simulink model "oldVers_1704_old1"  (R2022a)
settings: Solver=ode1  StartTime=0.0  StopTime=0.008  FixedStep=0.000001  RelTol=1e-3
values from neighbouring files (symbols this model uses):
  Cm = 0.05    [matlab2.mat]
  Jm = 1    [matlab2.mat]
  k_eq = 1    [matlab2.mat]
  k_pos = 1    [matlab2.mat]
  Ki_Curr = 1666    [matlab2.mat]
  Kinv = 18    [matlab2.mat]
  Kp_Curr = 0.0229017    [matlab2.mat]
  Re = 0.357267    [matlab2.mat]
  T_eq = 0.00052    [matlab2.mat]
  T_eq2 = 0.0018    [matlab2.mat]
  Te = 0.0006    [matlab2.mat]
  Tinv = 0.00026    [matlab2.mat]
undefined symbols (not defined in the file or in its folder): Kc_Curr, Kc_Pos, Kc_Speed
libraries: simulink x1
settings Model: Creator=Ruslan  LastModifiedBy=Ruslan
settings SolverCC: AlgebraicLoopSolver=TrustRegion
settings DebuggingCC: SFMachineParentedDataDiag=warning

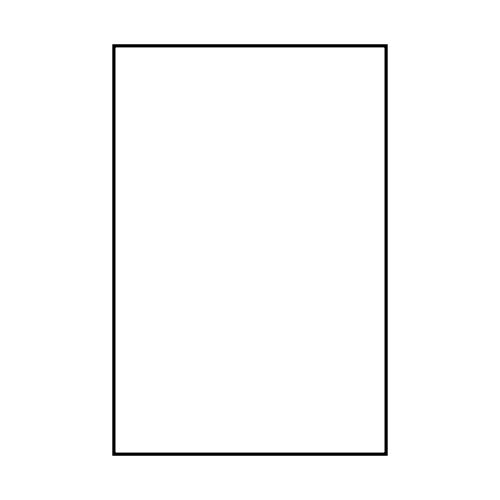
[thumbnail: Simulink's stored preview of the top-level diagram]
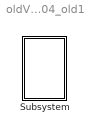
== system oldVers_1704_old1 ==
  Subsystem : Subsystem

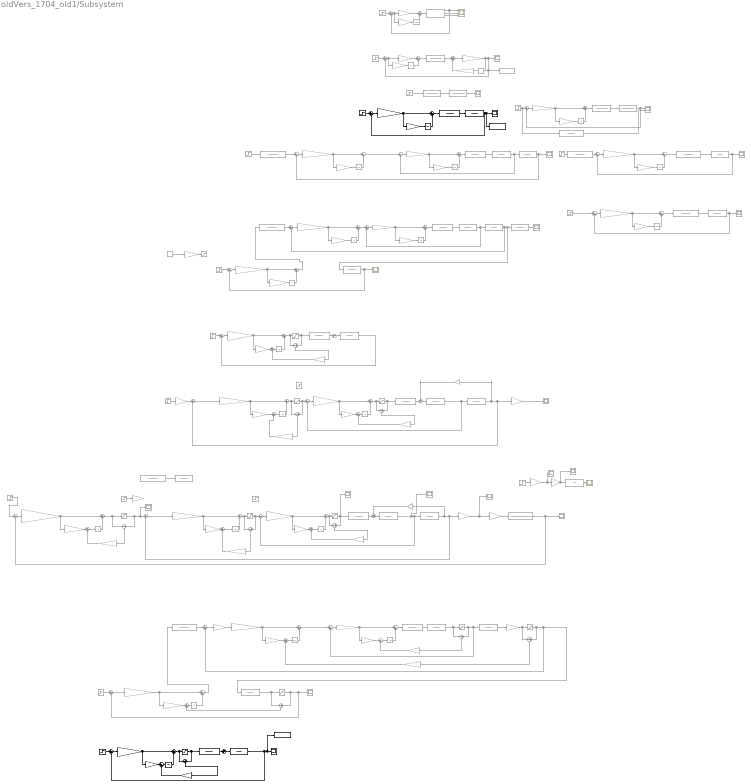
== system oldVers_1704_old1/Subsystem ==
  note: Рабочий Контур скорости с насыщениями
  note: Контур положения рабочий
  note: Контур скорости
  note: Контур тока
  note: Контур тока
  note: Контур тока рабочий
  1 : TransferFcn  Commented=on  Numerator=[Cm]  Denominator=[Jm 0]
  1/Rяц : Gain  Commented=on  Gain=1/0.357267
  {2..5} (4 alike) : TransferFcn  Commented=on  Numerator=[k_pos]  Denominator=[1 0]
  Derivative : Derivative  Commented=on
  Gain : Gain  Commented=on  Gain=Cm
  Gain1 : Gain  Commented=on  Gain=Cm
  Gain2 : Gain  Commented=on  Gain=k_pos*3.33333333333
  Integrator{,1,3..11,13..15,17,19..22} (19 alike) : Integrator  Commented=on
  Integrator12 : Integrator
  Integrator2 : Integrator
  Kп : Gain  Commented=on  Gain=0.00067
  Kп1 : Gain  Commented=on  Gain=0.00067
  Kп{4,7,10,14,17,30} (6 alike) : Gain  Commented=on  Gain=(Jm)/(2*T_eq*Cm)
  Kп11 : Gain  Commented=on  Gain=(1)/(2*T_eq2*k_pos)
  Kп12 : Gain  Commented=on  Gain=Te/(2*Tinv*Kinv*(1/Re))
  Kп13 : Gain  Commented=on  Gain=Kp_Curr
  Kп{15,18,20,26,31} (5 alike) : Gain  Commented=on  Gain=1/(30/pi)
  Kп16 : Gain  Commented=on  Gain=30/pi
  Kп19 : Gain  Commented=on  Gain=Te/(2*Tinv*Kinv*(1/Re))
  Kп2 : Gain  Commented=on  Gain=30/pi
  Kп21 : Gain  Gain=Te/(2*Tinv*Kinv*(1/Re))
  Kп25 : Gain  Commented=on  Gain=(0.06)/(2*T_eq2*k_pos*3.33333333333)
  Kп27 : Gain  Commented=on  Gain=(1)/(2*T_eq2*k_pos)
  Kп28 : Gain  Commented=on  Gain=Kp_Curr
  Kп29 : Gain  Commented=on  Gain=30/pi
  Kп3 : Gain  Commented=on  Gain=Kp_Curr
  Kп5 : Gain  Commented=on  Gain=0.0229017
  Kп6 : Gain  Commented=on  Gain=(1)/(2*T_eq2*k_pos)
  Kп8 : Gain  Gain=Te/(2*Tinv*Kinv*(1/Re))
  Kп9 : Gain  Commented=on  Gain=Te/(2*Tinv*Kinv*(1/Re))
  L : Gain  Commented=on  Gain=0.001457602
  Ramp1 : simulink/Sources/Ramp  Commented=on  slope=120  start=0  InitialOutput=0
  Saturation1 : Saturate  Commented=on  UpperLimit=96  LowerLimit=-40
  Saturation10 : Saturate  Commented=on  UpperLimit=91.6  LowerLimit=-91.6
  Saturation11 : Saturate  Commented=on  UpperLimit=70  LowerLimit=-70
  Saturation12 : Saturate  Commented=on  UpperLimit=1  LowerLimit=-1
  Saturation2 : Saturate  Commented=on  UpperLimit=70  LowerLimit=-70
  Saturation3 : Saturate  Commented=on  UpperLimit=1  LowerLimit=-1
  Saturation4 : Saturate  Commented=on  UpperLimit=1  LowerLimit=-1
  Saturation5 : Saturate  UpperLimit=1  LowerLimit=-1
  Saturation7 : Saturate  Commented=on  UpperLimit=70  LowerLimit=-70
  Saturation8 : Saturate  Commented=on  UpperLimit=750  LowerLimit=-750
  Saturation9 : Saturate  Commented=on  UpperLimit=900  LowerLimit=-900
  Scope : Scope  Commented=on  NumInputPorts=3
  Scope{1..2,4,6..19} (17 alike) : Scope  Commented=on
  Scope20 : Scope
  Scope3 : Scope
  Scope5 : Scope  Commented=on  NumInputPorts=2
  Step : Step  Commented=on  Time=0  After=-12  SampleTime=0
  Step{1..2,4..6,9,13..14} (8 alike) : Step  Commented=on  Time=0  SampleTime=0
  Step10 : Step  Commented=on  Time=0  After=875  SampleTime=0
  Step11 : Step  Commented=on  Time=0  After=96  SampleTime=0
  Step12 : Step  Commented=on  Time=0  After=875  SampleTime=0
  Step15 : Step  Commented=on  Time=0  After=70  SampleTime=0
  Step16 : Step  Commented=on  Time=0  After=18  SampleTime=0
  Step17 : Step  Time=0  After=10  SampleTime=0
  Step3 : Step  Time=0  SampleTime=0
  Step7 : Step  Commented=on  Time=0  After=140  SampleTime=0
  Step8 : Step  Commented=on  Time=0  After=85  SampleTime=0
  Sum{,2,8..9,12,15..16,20,24,27..28,31,35,39,43,51,55,57,61} (19 alike) : Sum  Commented=on  Inputs=|+-
  Sum{1,3,7,10..11,13..14,19,21,23,25..26,30,32,34,36,38,40,42,44,50,53..54,56,58,60,62,65} (28 alike) : Sum  Commented=on  Inputs=|++
  Sum17 : Sum  Commented=on  Inputs=-+|
  Sum18 : Sum  Commented=on  Inputs=-+|
  Sum{22,33,37,41,45,52,59,63..64} (9 alike) : Sum  Commented=on  Inputs=-|+
  Sum29 : Sum  Commented=on  Inputs=-+|
  Sum4 : Sum  Commented=on  Inputs=-+-
  Sum46 : Sum  Inputs=-+|
  Sum47 : Sum  Inputs=|++
  Sum48 : Sum  Inputs=|+-
  Sum49 : Sum  Inputs=|++
  Sum5 : Sum  Inputs=|++
  Sum6 : Sum  Inputs=|+-
  Sum66 : Sum  Inputs=-|+
  To Workspace : ToWorkspace  Commented=on  VariableName=simout  SaveFormat=Timeseries  SampleTime=-1
  To Workspace1 : ToWorkspace  VariableName=curr  SaveFormat=Timeseries  SampleTime=-1
  To Workspace2 : ToWorkspace  VariableName=curr2  SaveFormat=Timeseries  SampleTime=-1
  Аппроксимация ЗКС : TransferFcn  Commented=on  Denominator=[T_eq2 1]
  Аппроксимация ЗКС1 : TransferFcn  Commented=on  Denominator=[T_eq2 1]
  Аппроксимация ЗКТ : TransferFcn  Commented=on  Numerator=[k_eq]  Denominator=[T_eq 1]
  Аппроксимация ЗКТ1 : TransferFcn  Commented=on  Denominator=[T_eq 1]
  Аппроксимация ЗКТ3 : TransferFcn  Commented=on  Denominator=[4*T_eq 1]
  ДПТ : Subsystem  Commented=on
  Инвентор : TransferFcn  Commented=on  Numerator=[617.143]  Denominator=[0.00026 1]
  Инвентор1 : TransferFcn  Commented=on  Numerator=[18]  Denominator=[0.00026 1]
  Инвентор{3,5..8,10} (6 alike) : TransferFcn  Commented=on  Numerator=[Kinv]  Denominator=[Tinv 1]
  Инвентор2 : TransferFcn  Numerator=[Kinv]  Denominator=[Tinv 1]
  Инвентор4 : TransferFcn  Commented=on  Numerator=[18]  Denominator=[0.00026 1]
  Инвентор9 : TransferFcn  Numerator=[Kinv]  Denominator=[Tinv 1]
  Ки : Gain  Commented=on  Gain=0.22167
  Ки1 : Gain  Commented=on  Gain=0.22167
  Ки10 : Gain  Commented=on  Gain=Kc_Speed
  Ки11 : Gain  Commented=on  Gain=1/(4*T_eq2)
  Ки{8,12,17,28} (4 alike) : Gain  Commented=on  Gain=Kc_Curr
  Ки13 : Gain  Commented=on  Gain=1/Te
  Ки14 : Gain  Commented=on  Gain=Ki_Curr
  Ки{4,7,15,18,20,31} (6 alike) : Gain  Commented=on  Gain=1/(4*T_eq)
  Ки16 : Gain  Commented=on  Gain=1/k_pos
  Ки19 : Gain  Commented=on  Gain=Kc_Speed
  Ки2 : Gain  Gain=1/Te
  Ки21 : Gain  Commented=on  Gain=1/Te
  Ки22 : Gain  Gain=Kc_Curr
  Ки23 : Gain  Gain=1/Te
  Ки25 : Gain  Commented=on  Gain=0.05/(4*T_eq2)
  Ки26 : Gain  Commented=on  Gain=Kc_Pos
  Ки27 : Gain  Commented=on  Gain=1/(4*T_eq2)
  Ки29 : Gain  Commented=on  Gain=Ki_Curr
  Ки3 : Gain  Commented=on  Gain=Ki_Curr
  Ки30 : Gain  Commented=on  Gain=Kc_Speed
  Ки5 : Gain  Commented=on  Gain=1666
  Ки6 : Gain  Commented=on  Gain=1/(4*T_eq2)
  Ки9 : Gain  Commented=on  Gain=1/Te
  Оптимизирующее звено : TransferFcn  Commented=on  Denominator=[4*T_eq 1]
  Оптимизирующее звено3 : TransferFcn  Commented=on  Denominator=[4*T_eq 1]
  Оптимизирующий фильтр : TransferFcn  Commented=on  Denominator=[4*T_eq 1]
  мех сост{,1..3,5} (5 alike) : TransferFcn  Commented=on  Numerator=[Cm]  Denominator=[Jm 0]
  полож1 : TransferFcn  Commented=on  Numerator=[k_pos]  Denominator=[1 0]
  полож2 : TransferFcn  Commented=on  Numerator=[k_pos*3.33333333333]  Denominator=[1 0]
  полож3 : TransferFcn  Commented=on  Denominator=[1 0]
  электромагнит сост : TransferFcn  Commented=on  Numerator=[1/0.357267]  Denominator=[0.0006 1]
  электромагнит сост1 : TransferFcn  Numerator=[1/Re]  Denominator=[Te 1]
  электромагнит сост{2,4..7,9} (6 alike) : TransferFcn  Commented=on  Numerator=[1/Re]  Denominator=[Te 1]
  электромагнит сост3 : TransferFcn  Commented=on  Numerator=[1/0.357267]  Denominator=[0.0006 1]
  электромагнит сост8 : TransferFcn  Numerator=[1/Re]  Denominator=[Te 1]
  wires:
  Sum/1 -> Kп/1, Ки/1
  Sum1/1 -> ДПТ/1(Uвх)
  Ки/1 -> Integrator/1
  Step/1 -> Sum/1
  Kп/1 -> Sum1/1
  ДПТ/1(I) -> Sum/2, Scope/1
  ДПТ/3(M) -> Scope/3
  Integrator/1 -> Sum1/2
  ДПТ/2(ω) -> Scope/2
  Integrator1/1 -> Sum3/2
  Sum2/1 -> Kп1/1, Ки1/1
  Kп1/1 -> Sum3/1
  Ки1/1 -> Integrator1/1
  Step1/1 -> Sum2/1
  Sum4/1 -> 1/Rяц/1
  L/1 -> Sum4/3
  Derivative/1 -> L/1
  1/Rяц/1 -> Derivative/1, To Workspace/1, Sum2/2, Scope2/1  "Iя"
  Sum3/1 -> Инвентор/1
  Инвентор/1 -> Sum4/2
  Step2/1 -> Инвентор1/1
  Инвентор1/1 -> электромагнит сост/1
  электромагнит сост/1 -> Scope1/1
  Инвентор2/1 -> электромагнит сост1/1
  электромагнит сост1/1 -> Scope3/1, To Workspace1/1, Sum6/2
  Ки2/1 -> Integrator2/1
  Integrator2/1 -> Sum5/2
  Kп8/1 -> Ки2/1, Sum5/1
  Sum5/1 -> Инвентор2/1
  Step3/1 -> Sum6/1
  Sum6/1 -> Kп8/1
  Kп3/1 -> Sum7/1, Ки3/1
  Integrator3/1 -> Sum7/2
  Sum8/1 -> Kп3/1
  электромагнит сост2/1 -> мех сост/1, Sum8/2
  Инвентор3/1 -> электромагнит сост2/1
  Sum7/1 -> Инвентор3/1  "выход регулятора тока в КОНТУРЕ СКОРОСТИ без насыщений"
  Ки3/1 -> Integrator3/1
  Kп4/1 -> Ки4/1, Sum10/1
  Integrator4/1 -> Sum10/2
  Ки4/1 -> Integrator4/1
  Sum9/1 -> Kп4/1
  Sum10/1 -> Sum8/1  "выход регулятора скорости без насыщений"
  мех сост/1 -> Sum9/2, Scope4/1  "ОС КОНТУР СКОРОСТИ без насыщений"
  Kп5/1 -> Sum11/1, Ки5/1
  Integrator5/1 -> Sum11/2
  Sum12/1 -> Kп5/1
  Step5/1 -> Аппроксимация ЗКТ/1, Sum12/1
  электромагнит сост3/1 -> Scope5/1, Sum12/2
  Инвентор4/1 -> электромагнит сост3/1
  Sum11/1 -> Инвентор4/1
  Ки5/1 -> Integrator5/1
  Аппроксимация ЗКТ/1 -> Scope5/2
  Ки7/1 -> Integrator7/1
  Sum13/1 -> Аппроксимация ЗКТ1/1
  Kп7/1 -> Ки7/1, Sum13/1
  Sum16/1 -> Kп7/1
  Аппроксимация ЗКТ1/1 -> 1/1
  Integrator7/1 -> Sum13/2
  1/1 -> Scope6/1, Sum16/2
  Step6/1 -> Аппроксимация ЗКТ3/1
  Аппроксимация ЗКТ3/1 -> Sum16/1
  Step4/1 -> Оптимизирующий фильтр/1
  Оптимизирующий фильтр/1 -> Sum9/1
  2/1 -> Scope9/1, Sum15/2
  Sum14/1 -> Аппроксимация ЗКС/1
  Ки6/1 -> Integrator6/1
  Kп6/1 -> Ки6/1, Sum14/1
  Sum15/1 -> Kп6/1
  Integrator6/1 -> Sum14/2
  Step9/1 -> Sum15/1
  Аппроксимация ЗКС/1 -> 2/1
  Kп11/1 -> Ки11/1, Sum23/1
  Sum24/1 -> Kп11/1
  Sum23/1 -> Оптимизирующее звено/1  "Выход с регулятора положения без насыщений"
  3/1 -> Scope8/1, Sum24/2  "КП реакция на ступеньку без насыщений"
  Integrator11/1 -> Sum23/2
  Ки11/1 -> Integrator11/1
  мех сост1/1 -> Sum28/2, 3/1, полож1/1
  Sum28/1 -> Kп14/1
  Инвентор5/1 -> электромагнит сост4/1
  электромагнит сост4/1 -> мех сост1/1, Sum27/2
  Kп14/1 -> Ки15/1, Sum25/1
  Ки14/1 -> Integrator13/1
  Integrator13/1 -> Sum26/2
  Sum26/1 -> Инвентор5/1
  Sum27/1 -> Kп13/1
  Kп13/1 -> Sum26/1, Ки14/1
  Integrator14/1 -> Sum25/2
  Sum25/1 -> Sum27/1  "КОНТУР ПОЛОЖЕНИЯ выход регулятора скорости БЕЗ насыщения"
  полож1/1 -> Scope12/1
  Ки15/1 -> Integrator14/1
  Ки16/1 -> Saturation1/1
  Ramp1/1 -> Ки16/1
  Оптимизирующее звено/1 -> Sum28/1
  Ки17/1 -> Sum36/2
  Ки9/1 -> Sum36/1
  Sum36/1 -> Integrator15/1
  Sum34/1 -> Sum37/1, Saturation12/1
  Sum35/1 -> Kп9/1
  Kп9/1 -> Ки9/1, Sum34/1
  Integrator15/1 -> Sum34/2
  Sum37/1 -> Ки17/1
  электромагнит сост6/1 -> мех сост3/1, Sum35/2  "ВЫХОД КОНТУРА ТОКА"
  Sum38/1 -> Sum41/1, Saturation11/1
  Kп17/1 -> Ки20/1, Sum38/1
  Integrator17/1 -> Sum38/2
  Sum40/1 -> Integrator17/1
  Ки20/1 -> Sum40/1
  мех сост3/1 -> Kп16/1, Sum39/2, Gain/1  "ОС КОНТУР СКОРОСТИ с насыщениями"
  Sum39/1 -> Kп17/1
  Ки19/1 -> Sum40/2
  Sum41/1 -> Ки19/1
  Sum51/1 -> Kп25/1
  Step11/1 -> Sum51/1
  Kп25/1 -> Sum50/1, Ки25/1
  полож2/1 -> Scope14/1, Sum51/2  "КП реакция на ступеньку с насыщениями"
  Ки25/1 -> Sum53/1
  Sum53/1 -> Integrator19/1
  Ки26/1 -> Sum53/2
  Kп26/1 -> полож2/1
  Step12/1 -> Kп18/1
  Sum50/1 -> Sum52/1, Saturation10/1
  Step13/1 -> Sum24/1
  Step14/1 -> Sum55/1
  Sum55/1 -> Kп27/1
  Kп27/1 -> Sum54/1, Ки27/1
  Integrator20/1 -> Sum54/2
  Saturation8/1 -> Sum63/2, 4/1, Sum61/2
  Sum63/1 -> Ки30/1
  электромагнит сост9/1 -> Sum59/1, Saturation7/1
  Инвентор10/1 -> электромагнит сост9/1
  Ки28/1 -> Sum58/2
  Sum59/1 -> Ки28/1
  Sum61/1 -> Kп31/1
  Kп30/1 -> Ки31/1, Sum60/1
  Ки31/1 -> Sum62/1
  Оптимизирующее звено3/1 -> Sum61/1
  Sum62/1 -> Integrator22/1
  Sum60/1 -> Sum57/1
  Kп29/1 -> Sum63/1, Saturation8/1
  Integrator21/1 -> Sum56/2
  Integrator22/1 -> Sum60/2
  мех сост5/1 -> Kп29/1
  Kп31/1 -> Kп30/1
  Saturation7/1 -> Sum59/2, мех сост5/1, Sum57/2
  Sum57/1 -> Kп28/1
  Sum58/1 -> Integrator21/1
  Sum56/1 -> Инвентор10/1
  Sum54/1 -> Оптимизирующее звено3/1
  Kп28/1 -> Ки29/1, Sum56/1
  Ки29/1 -> Sum58/1
  Ки30/1 -> Sum62/2
  Sum64/1 -> Sum65/2
  4/1 -> Sum64/1, Saturation9/1
  Saturation9/1 -> Sum64/2, Sum55/2, Scope16/1
  Ки27/1 -> Sum65/1
  Sum65/1 -> Integrator20/1
  Saturation12/1 -> Sum37/2, Инвентор7/1  "Выход регулятора тока в КОНТУРЕ СКОРОСТИ с насыщениями"
  Saturation11/1 -> Sum41/2, Sum35/1  "Выход регулятора скорости с насыщениями"
  Инвентор7/1 -> Sum17/2
  Sum17/1 -> электромагнит сост6/1
  Gain/1 -> Sum17/1
  Saturation10/1 -> Scope19/1, Sum43/1, Sum52/2  "выход регулятор положения"
  Saturation2/1 -> Sum20/1, Sum45/2  "Выход регулятора скорости с насыщениями"
  Saturation3/1 -> Scope10/1, Sum22/2, Инвентор6/1  "Выход регулятора тока в КОНТУРЕ СКОРОСТИ с насыщениями"
  Sum45/1 -> Ки10/1
  Инвентор6/1 -> Sum18/2
  Kп10/1 -> Ки18/1, Sum42/1
  Sum22/1 -> Ки8/1
  Sum20/1 -> Kп19/1
  Sum21/1 -> Integrator8/1
  мех сост2/1 -> Kп2/1, Sum43/2, Gain1/1  "ОС КОНТУР СКОРОСТИ с насыщениями"
  Sum44/1 -> Integrator9/1
  Sum18/1 -> электромагнит сост5/1
  Ки18/1 -> Sum44/1
  электромагнит сост5/1 -> Scope11/1, мех сост2/1, Sum20/2  "ВЫХОД КОНТУРА ТОКА"
  Sum19/1 -> Sum22/1, Saturation3/1
  Integrator8/1 -> Sum19/2
  Ки10/1 -> Sum44/2
  Sum43/1 -> Kп10/1
  Ки21/1 -> Sum21/1
  Sum42/1 -> Sum45/1, Saturation2/1
  Ки8/1 -> Sum21/2
  Kп19/1 -> Ки21/1, Sum19/1
  Integrator9/1 -> Sum42/2
  Инвентор8/1 -> Sum29/2
  Sum29/1 -> электромагнит сост7/1
  Step8/1 -> Sum31/1  "Выход регулятора скорости с насыщениями"
  Ки13/1 -> Sum32/1
  Saturation4/1 -> Sum33/2, Инвентор8/1  "Выход регулятора тока в КОНТУРЕ СКОРОСТИ с насыщениями"
  Sum33/1 -> Ки12/1
  Sum31/1 -> Kп12/1
  Sum32/1 -> Integrator10/1
  Integrator10/1 -> Sum30/2
  электромагнит сост7/1 -> Sum31/2  "ВЫХОД КОНТУРА ТОКА"
  Ки12/1 -> Sum32/2
  Kп12/1 -> Ки13/1, Sum30/1
  Sum30/1 -> Sum33/1, Saturation4/1
  Аппроксимация ЗКС1/1 -> 5/1
  Gain1/1 -> Sum18/1
  Step16/1 -> Kп20/1  "ОС КОНТУР СКОРОСТИ с насыщениями"
  Kп20/1 -> Scope18/1, Gain2/1
  полож3/1 -> Scope15/1  "КП реакция на ступеньку с насыщениями"
  Gain2/1 -> полож3/1, Scope17/1
  Kп16/1 -> Scope13/1  "ОС КОНТУР СКОРОСТИ с насыщениями"
  Kп18/1 -> Sum39/1
  Step10/1 -> Kп15/1
  Kп2/1 -> Scope7/1, Kп26/1  "ОС КОНТУР СКОРОСТИ с насыщениями"
  Integrator19/1 -> Sum50/2
  Sum52/1 -> Ки26/1
  Integrator12/1 -> Sum47/2
  электромагнит сост8/1 -> To Workspace2/1, Scope20/1, Sum48/2  "ВЫХОД КОНТУРА ТОКА"
  Sum48/1 -> Kп21/1
  Инвентор9/1 -> Sum46/2
  Saturation5/1 -> Sum66/2, Инвентор9/1  "Выход регулятора тока в КОНТУРЕ СКОРОСТИ с насыщениями"
  Ки23/1 -> Sum49/1
  Step17/1 -> Sum48/1  "Выход регулятора скорости с насыщениями"
  Sum66/1 -> Ки22/1
  Sum46/1 -> электромагнит сост8/1
  Sum47/1 -> Sum66/1, Saturation5/1
  Sum49/1 -> Integrator12/1
  Kп21/1 -> Ки23/1, Sum47/1
  Ки22/1 -> Sum49/2

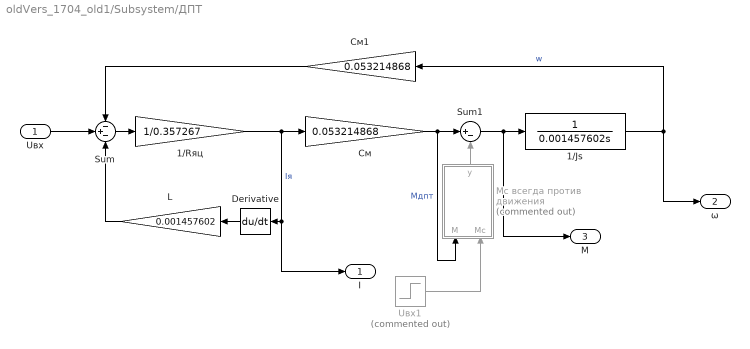
== system oldVers_1704_old1/Subsystem/ДПТ ==
  Uвх : Inport
  1/Js : TransferFcn  Denominator=[0.001457602 0]
  1/Rяц : Gain  Gain=1/0.357267
  Cм : Gain  Gain=0.053214868
  Cм1 : Gain  Gain=0.053214868
  Derivative : Derivative
  L : Gain  Gain=0.001457602
  Sum : Sum  Inputs=-+-
  Sum1 : Sum  Inputs=|+-
  Uвх1 : Step  Commented=on  After=0.06  SampleTime=0
  Мс всегда против движения : MATLAB Function  Commented=on  TreatAsAtomicUnit=on
  I : Outport
  ω : Outport  Port=2
  M : Outport  Port=3
  wires:
  1/Rяц/1 -> I/1, Derivative/1, Cм/1  "Iя"
  Uвх/1 -> Sum/2
  L/1 -> Sum/3
  1/Js/1 -> Cм1/1, ω/1  "w"
  Cм1/1 -> Sum/1
  Derivative/1 -> L/1
  Sum1/1 -> M/1, 1/Js/1
  Uвх1/1 -> Мс всегда против движения/2(Mc)
  Sum/1 -> 1/Rяц/1
  Cм/1 -> Мс всегда против движения/1(M), Sum1/1  "Мдпт"
  Мс всегда против движения/1(y) -> Sum1/2

== matlab function oldVers_1704_old1/Subsystem/ДПТ/Мс всегда против движения ==
  data: M input; Mc input; y output
function y = fcn(M, Mc)
if (M>0)
    y = Mc;
else
    y = -Mc;
end
